simulink model "controllhybrid"  (R2021b)
settings: Solver=ode1  StartTime=0  StopTime=10  FixedStep=0.01  RelTol=1e-3
settings Model: Creator=hukai  LastModifiedBy=hukai

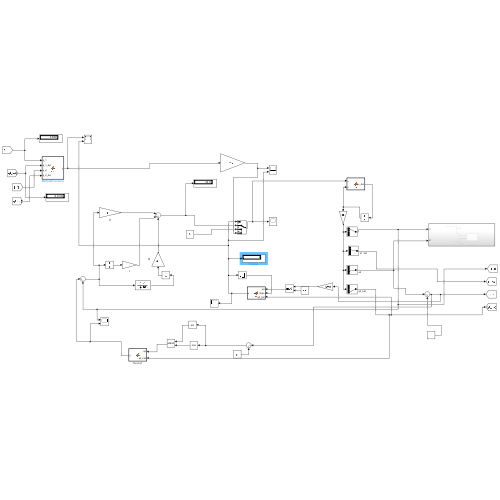
[thumbnail: Simulink's stored preview of the top-level diagram]
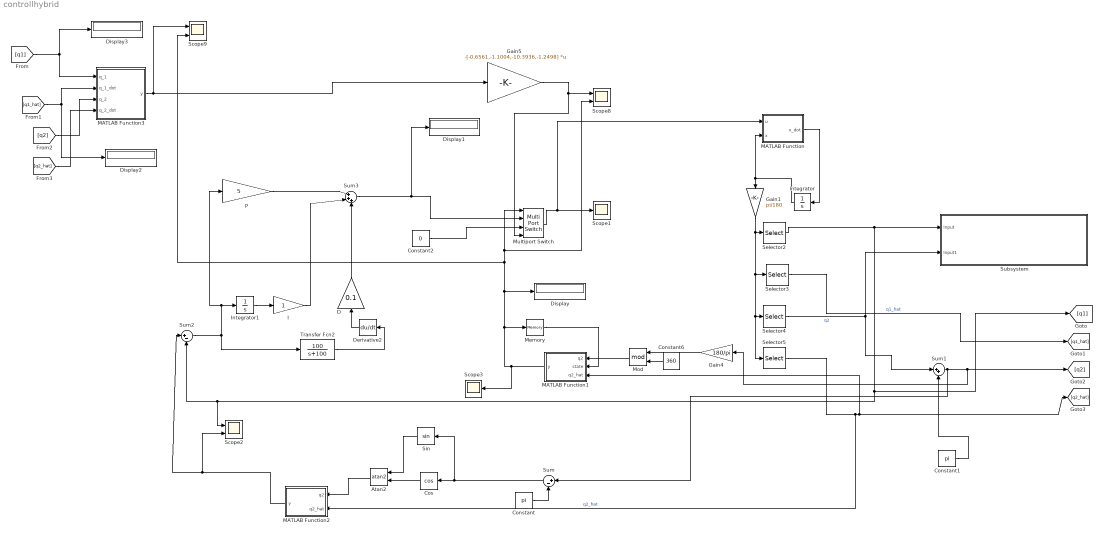
== system controllhybrid ==
  Atan2 : Trigonometry  Operator=atan2
  Constant : Constant  Value=pi
  Constant1 : Constant  Value=pi
  Constant2 : Constant  Value=0
  Constant6 : Constant  Value=360
  Cos : Trigonometry  Operator=cos
  D : Gain  Gain=0.1
  Derivative2 : Derivative
  Display{,1..3} (4 alike) : Display
  Gain1 : Gain  Gain=pi/180
  Gain4 : Gain  Gain=180/pi
  Gain5 : Gain  Gain=-[-0.6561,-1.1004,-10.3936,-1.2498]  Multiplication=Matrix(K*u)
  I : Gain
  Integrator : Integrator  InitialCondition=[0;0;20;0]
  Integrator1 : Integrator
  MATLAB Function : MATLAB Function  TreatAsAtomicUnit=on
  MATLAB Function1 : MATLAB Function  TreatAsAtomicUnit=on
  MATLAB Function2 : MATLAB Function  Tag=Desired  TreatAsAtomicUnit=on
      settings: AttributesFormatString=%<Tag>
  MATLAB Function3 : MATLAB Function  TreatAsAtomicUnit=on
  Memory : Memory  InitialCondition=1
  Mod : Math  Operator=mod  SaturateOnIntegerOverflow=on
  Multiport Switch : MultiPortSwitch
  P : Gain  Gain=5
  Scope1 : Scope
  Scope2 : Scope  NumInputPorts=2
  Scope3 : Scope
  Scope8 : Scope  NumInputPorts=2
  Scope9 : Scope  NumInputPorts=2
  Selector2 : Selector  InputPortWidth=4  IndexOptions=Index vector (dialog)  Indices=1  OutputSizes=1
  Selector3 : Selector  InputPortWidth=4  IndexOptions=Index vector (dialog)  Indices=2  OutputSizes=1
  Selector4 : Selector  InputPortWidth=4  IndexOptions=Index vector (dialog)  Indices=3  OutputSizes=1
  Selector5 : Selector  InputPortWidth=4  IndexOptions=Index vector (dialog)  Indices=4  OutputSizes=1
  Sin : Trigonometry
  Subsystem : Subsystem
  Sum : Sum  Inputs=|+-
  Sum1 : Sum  Inputs=|++
  Sum2 : Sum  Inputs=|+-
  Sum3 : Sum  Inputs=|+++
  Transfer Fcn2 : TransferFcn  Numerator=100  Denominator=[1 100]
  wires:
  MATLAB Function/1(x_dot) -> Integrator/1
  Integrator/1 -> Gain1/1, MATLAB Function/2(x)
  Atan2/1 -> MATLAB Function2/1(q2)
  [q1] -> Display3/1, MATLAB Function3/1(q_1)
  Constant2/1 -> Multiport Switch/3
  Gain5/1 -> Multiport Switch/4, Scope8/1
  MATLAB Function3/1(y) -> Scope9/1, Gain5/1
  [q2_hat] -> MATLAB Function3/4(q_2_dot)
  Cos/1 -> Atan2/2
  [q1_hat] -> Display2/1, MATLAB Function3/2(q_1_dot)
  [q2] -> MATLAB Function3/3(q_2)
  D/1 -> Sum3/3
  MATLAB Function1/1(y) -> Scope3/1, Memory/1, Scope9/2, Scope8/2, Multiport Switch/1, Display/1
  Sum3/1 -> Display1/1, Multiport Switch/2
  Sin/1 -> Atan2/1
  Sum2/1 -> P/1, Integrator1/1, Transfer Fcn2/1
  Transfer Fcn2/1 -> Derivative2/1
  P/1 -> Sum3/1
  Derivative2/1 -> D/1
  Memory/1 -> MATLAB Function1/2(state)
  I/1 -> Sum3/2
  Integrator1/1 -> I/1
  Selector4/1 -> Sum1/1, Subsystem/2(Input1)  "q2"
  Selector2/1 -> Scope2/1, Sum2/2, [q1], Subsystem/1(Input)
  Selector3/1 -> [q1_hat]  "q1_hat"
  Selector5/1 -> MATLAB Function2/2(q2_hat), [q2_hat], MATLAB Function1/3(q2_hat)  "q2_hat"
  Sum/1 -> Sin/1, Cos/1
  Gain4/1 -> Mod/1
  Constant6/1 -> Mod/2
  Mod/1 -> MATLAB Function1/1(q2)
  Constant/1 -> Sum/2
  Sum1/1 -> Sum/1, Gain4/1, [q2]
  Constant1/1 -> Sum1/2
  MATLAB Function2/1(y) -> Scope2/2, Sum2/1
  Multiport Switch/1 -> MATLAB Function/1(u), Scope1/1
  Gain1/1 -> Selector5/1, Selector4/1, Selector3/1, Selector2/1

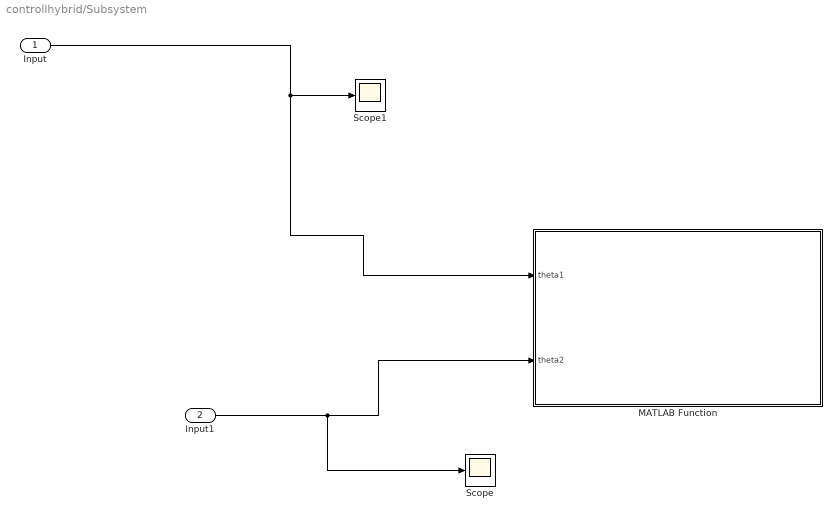
== system controllhybrid/Subsystem ==
  Input : Inport
  Input1 : Inport  Port=2
  MATLAB Function : MATLAB Function  TreatAsAtomicUnit=on
  Scope : Scope
  Scope1 : Scope
  wires:
  Input/1 -> MATLAB Function/1(theta1), Scope1/1
  Input1/1 -> Scope/1, MATLAB Function/2(theta2)

== matlab function controllhybrid/MATLAB Function ==
  data: u input; x_dot output; x input
function x_dot  = fcn(u, x)

theta_1_dot = 0.0171;
theta_2_dot = 0.0038;
theta_3_dot = 0.0038;
theta_4_dot = 0.0921;

theta_1 = 0.0304;
theta_2 = 0.0184;
theta_3 = 0.0184;
theta_4 = 0.0921;
theta_5 = 0.6101;
theta_6 = 0.0097;

q_1 = x(1);
q_1_dot = x(2);
q_2= x(3);
q_2_dot=x(4);
q_dot = [q_1_dot;q_2_dot];

m_11 = theta_1+theta_2*sin(q_2)^2;
m_12 = theta_3*cos(q_2);
c_11 = 2*theta_2*sin(q_2)*cos(q_2)*q_2_dot;
c_12 = -theta_3*sin(q_2)*q_2_dot;
f_1 = theta_5*q_1_dot;
g_1 = 0;

m_21 = theta_3*cos(q_2);
m_22 = theta_2;
c_21 = -theta_2*sin(q_2)*cos(q_2)*q_1_dot;
c_22 = 0;
f_2 = theta_6*q_2_dot;
g_2 = 9.8*-theta_4*sin(q_2);

M = [m_11,m_12;m_21,m_22];
C = [c_11,c_12;c_21,c_22];
F = [f_1;f_2];
G = [g_1;g_2];
q_ddot = M^(-1)*(u-C*q_dot-F-G);
q_1_ddot = q_ddot(1);
q_2_ddot = q_ddot(2);
x_dot = [q_1_dot;
         q_1_ddot;
         q_2_dot;
         q_2_ddot;];

== matlab function controllhybrid/Subsystem/MATLAB Function ==
  data: theta1 input; theta2 input
function  fcn(theta1,theta2)
link1_frame1 = [0,0,0;
                0,0,-1;
                0,6,-1;
                0,6,0;
                0,8,0]; % declaration of link1 points in FRAME-1
link1_frame0 = zeros(5,3);
link2_frame2 = [0,0,0;
                0,12,0]; % declaration of link2 points in FRAME-1    
link2_frame1 = zeros(2,3);
link2_frame0 = zeros(2,3);
plot3([0,0],[0,0],[-10,0],'ks-','LineWidth',1) % drawing of robot base in FRAME-0
hold on
for i = 1:length(link1_frame1(:,1))
    link1_frame0(i,:) = TRANS0_1(link1_frame1(i,:),theta1); 
    % transformation of link1 points from FRAME-1 to FRAME-0
end
plot3(link1_frame0(:,1),link1_frame0(:,2),link1_frame0(:,3),'bs-','LineWidth',1)
for i = 1:length(link2_frame2(:,1))
    link2_frame1(i,:) = TRANS1_2(link2_frame2(i,:),theta2,6,2);
    link2_frame0(i,:) = TRANS0_1(link2_frame1(i,:),theta1);
end
plot3(link2_frame0(:,1),link2_frame0(:,2),link2_frame0(:,3),'rs-','LineWidth',1)
hold off
grid on
axis([-15 15 -15 15 -15 15])
title('Drawing of Base and Links 1-2 in FRAME-0 animating') 
pause(0.001)

function fr0 = TRANS0_1(fr1, theta1)
fr1_cat = cat(2,fr1,1)';
% creates a usable 4-vector by concatination and transpose
T0_1 = [cos(theta1),-sin(theta1),0,0;
        sin(theta1),cos(theta1),0,0;
        0,0,1,0;
        0,0,0,1];
fr0_cat = (T0_1*fr1_cat);
fr0 = fr0_cat(1:3)';
end

function fr1 = TRANS1_2(fr2, theta2, l1, l2)
fr2_cat = cat(2,fr2,1)';
% creates a usable 4-vector by concatination and transpose
T1_2 = [cos(theta2),-sin(theta2),0,0;
        0,0,-1,l1+l2;
        sin(theta2),cos(theta2),0,0;
        0,0,0,1];
fr1_cat = (T1_2*fr2_cat);
fr1 = fr1_cat(1:3)';
end
% drawing link2 points and segments in FRAME-0

end

== matlab function controllhybrid/MATLAB Function1 ==
  data: q2 input; y output; state input; q2_hat input
function y = fcn(q2,state,q2_hat)
% in state 1
if (q2 > 170) && (q2 < 190) && (state == 2) &&(abs(q2_hat)<0.5)
    y = 1;
elseif ((q2 < 20) && (q2 >0) && (state ==1)) || ((q2 >340) && (q2 <360) && (state ==1))
    y = 3;
elseif ((q2 > 20) && (state ==3))&& (q2 < 340)
    y = 2;
else 
    y =state;
end

%atan(sin(q2), cos(q2))

== matlab function controllhybrid/MATLAB Function2 ==
  data: q2 input; y output; q2_hat input
function y = fcn(q2,q2_hat)
k1 = 1;
k2 = 0;
y = k1*q2+k2*q2_hat;

== matlab function controllhybrid/MATLAB Function3 ==
  data: y output; q_1 input; q_1_dot input; q_2 input; q_2_dot input
function y = fcn(q_1,q_1_dot,q_2,q_2_dot)
q_2 = atan2(sin(q_2),cos(q_2));
q_hat = [q_1;q_1_dot;q_2;q_2_dot];
y = q_hat;
